simulink model "test_td"  (R2022b)
settings: Solver=VariableStepAuto  StartTime=0.0  StopTime=10  RelTol=1e-3
undefined symbols (not defined in the file or in its folder): den, num
libraries: simulink x2, slpidlib x1, dspsrcs4 x1
settings Model: Creator=张倬境  LastModifiedBy=张倬境

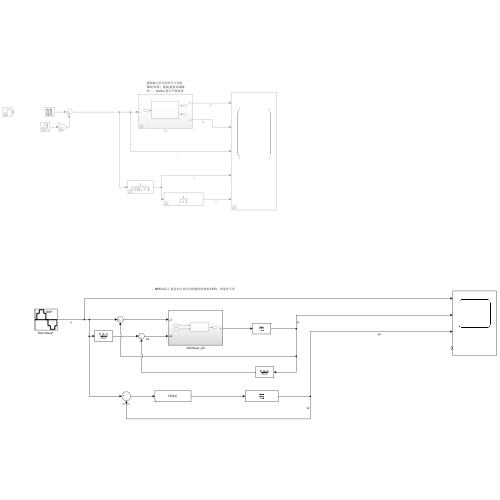
[thumbnail: Simulink's stored preview of the top-level diagram]
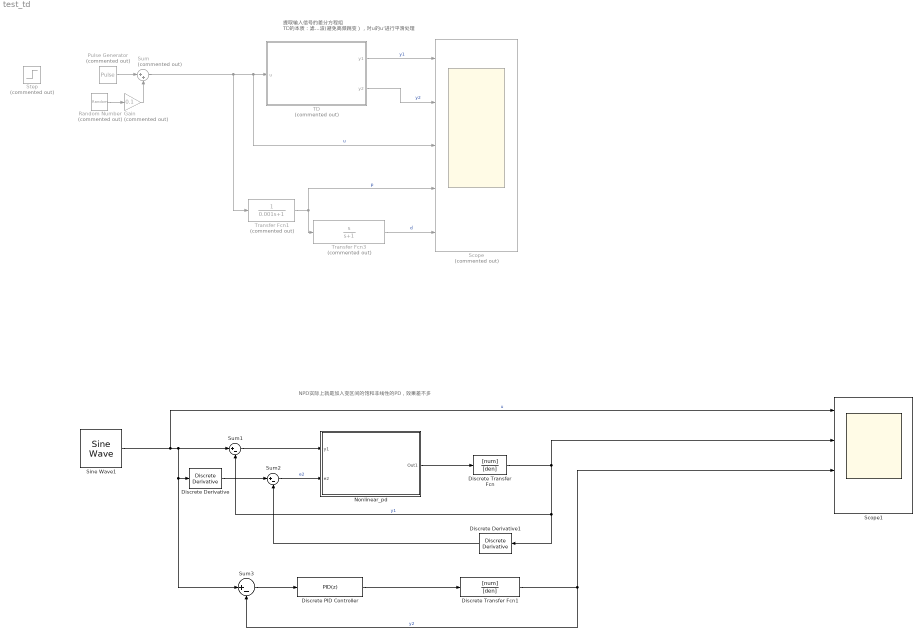
== system test_td ==
  note: NPD实际上就是加入变区间的饱和非线性的PD，效果差不多
  note: 提取输入信号的差分方程组
      | TD的本质：滤波(避免高频跳变），对u的u‘进行平滑处理
  Discrete Transfer Fcn : DiscreteTransferFcn  Numerator=[num]  Denominator=[den]
  Discrete Transfer Fcn1 : DiscreteTransferFcn  Numerator=[num]  Denominator=[den]
  Discrete Derivative : simulink/Discrete/Discrete Derivative  gainval=1.0  ICPrevScaledInput=0.0  OutMin=[]  OutMax=[]  OutDataType=fixdt(1, 16)  OutScaling=2^-10  DoSatur=off
  Discrete Derivative1 : simulink/Discrete/Discrete Derivative  gainval=1.0  ICPrevScaledInput=0.0  OutMin=[]  OutMax=[]  OutDataType=fixdt(1, 16)  OutScaling=2^-10  DoSatur=off
  Discrete PID Controller : slpidlib/PID Controller  Controller=PID  Form=Parallel  TimeDomain=Discrete-time  UseExternalTs=off  SampleTime=-1  IntegratorMethod=Forward Euler  FilterMethod=Forward Euler  ControllerParametersSource=internal  P=100  I=0  UseKiTs=off  D=0  N=10  UseFilter=off  TunerSelectOption=Frequency Response Based  InitialConditionSource=internal  InitialConditionForIntegrator=0  InitialConditionForFilter=0  DifferentiatorICPrevScaledInput=0  ExternalReset=none  TrackingMode=off  Kt=1  LimitOutput=off  SatLimitsSource=internal  UpperSaturationLimit=inf  LowerSaturationLimit=-inf  LinearizeAsGain=off  AntiWindupMode=none  Kb=1  LimitIntegrator=off  UpperIntegratorSaturationLimit=inf  LowerIntegratorSaturationLimit=-inf  POutMin=[]  POutMax=[]  IOutMin=[]  IOutMax=[]  DOutMin=[]  DOutMax=[]  NOutMin=[]  NOutMax=[]  SumOutMin=[]  SumOutMax=[]  SaturationOutMin=[]  SaturationOutMax=[]  PParamMin=[]  PParamMax=[]  IParamMin=[]  IParamMax=[]  DParamMin=[]  DParamMax=[]  NParamMin=[]  NParamMax=[]  KbParamMin=[]  KbParamMax=[]  KtParamMin=[]  KtParamMax=[]  KbOutMin=[]  KbOutMax=[]  KtOutMin=[]  KtOutMax=[]  IntegratorOutMin=[]  IntegratorOutMax=[]  FilterOutMin=[]  FilterOutMax=[]  SumI1OutMin=[]  SumI1OutMax=[]  SumI2OutMin=[]  SumI2OutMax=[]  SumI3OutMin=[]  SumI3OutMax=[]  SumI4OutMin=[]  SumI4OutMax=[]  SumDOutMin=[]  SumDOutMax=[]  DifferentiatorOutMin=[]  DifferentiatorOutMax=[]  FilterDiffOutCoefMin=[]  FilterDiffOutCoefMax=[]  ReciprocalOutMin=[]  ReciprocalOutMax=[]  SumDenOutMin=[]  SumDenOutMax=[]  SumNumOutMin=[]  SumNumOutMax=[]  DivideOutMin=[]  DivideOutMax=[]  UdiffTsProdOutMin=[]  UdiffTsProdOutMax=[]  NTsProdOutMin=[]  NTsProdOutMax=[]  UintegralTsProdOutMin=[]  UintegralTsProdOutMax=[]  UngainTsProdOutMin=[]  UngainTsProdOutMax=[]  ClampingZeroOutDataTypeStr=Inherit: Inherit via back propagation  ClampingZeroOutMin=[]  ClampingZeroOutMax=[]  FilterDenConstantOutDataTypeStr=Inherit: Inherit via back propagation  FilterDenConstantOutMin=[]  FilterDenConstantOutMax=[]  PCopyOutDataTypeStr=Inherit: Inherit via back propagation  PCopyOutMin=[]  PCopyOutMax=[]  NCopyOutDataTypeStr=Inherit: Inherit via back propagation  NCopyOutMin=[]  NCopyOutMax=[]  IntegratorContinuousStateAttributes=''  IntegratorStateMustResolveToSignalObject=off  IntegratorRTWStateStorageClass=Auto  FilterContinuousStateAttributes=''  FilterStateMustResolveToSignalObject=off  FilterRTWStateStorageClass=Auto  ParallelPVariant=InternalParameters  IdealPVariant=Disabled  IVariant=InternalParameters  DVariant=InternalParameters  IntegratorVariant=Discrete  SatVariant=Disabled  AWVariant=Passthrough  PCopyVariant=Disabled  TRVariant=Disabled  FdbkBlocksVariant=Forward  IdealPFdbkVariant=Disabled  SatFdbkVariant=Disabled  DerivativeFilterVariant=Differentiator  NVariant=Passthrough  NCopyVariant=Disabled_SignalSpec  FilterICVariant=InternalICsDifferentiator  IntegratorICVariant=InternalICs  ExternalResetVariant=Disabled  TRSumVariant=Passthrough  SumFdbkVariant=Disabled  SumVariant=Sum_PID  TsampFilterVariant=InternalTs  TsampNgainVariant=Passthrough  TsampIntegralVariant=Passthrough  ExternalSaturationOutDataTypeStr=Inherit: Same as second input
      settings: LibrarySourceBlock=simulink/Discrete/Discrete PID Controller
  Gain : Gain  Commented=on  Gain=0.1
  Nonlinear_pd : Subsystem
  Pulse Generator : DiscretePulseGenerator  Commented=on  PulseType=Time based  Period=4  PulseWidth=50
  Random Number : RandomNumber  Commented=on  Variance=0.01  SampleTime=0.1
  Scope : Scope  Commented=on  NumInputPorts=5
  Scope1 : Scope  NumInputPorts=4
  Sine Wave1 : dspsrcs4/Sine Wave  Amplitude=1  Frequency=1/4  Phase=0  SampleMode=Discrete  OutComplex=Real  CompMethod=Trigonometric fcn  TableSize=Speed  SampleTime=1/100  SamplesPerFrame=1  ResetState=Restart at time zero  OutputFrames=off  dataType=double  wordLen=16  udDataType=sfix(16)  fracBitsMode=Best precision  numFracBits=15  OutDataTypeStr=double  LastOutDataTypeStr=double
  Step : Step  Commented=on  SampleTime=0
  Sum : Sum  Commented=on  Inputs=|++
  Sum1 : Sum  Inputs=|+-
  Sum2 : Sum  Inputs=|+-
  Sum3 : Sum  Inputs=|+-
  TD : Subsystem  Commented=on
  Transfer Fcn1 : TransferFcn  Commented=on  Denominator=[0.001 1]
  Transfer Fcn3 : TransferFcn  Commented=on  Numerator=[1 0]  Denominator=[1 1]
  wires:
  Sum/1 -> Transfer Fcn1/1, Scope/3, TD/1(u)  "u"
  Random Number/1 -> Gain/1
  Gain/1 -> Sum/2
  TD/1(y1) -> Scope/1  "y1"
  Transfer Fcn1/1 -> Scope/4, Transfer Fcn3/1  "p"
  TD/2(y2) -> Scope/2  "y2"
  Transfer Fcn3/1 -> Scope/5  "d"
  Pulse Generator/1 -> Sum/1
  Sum1/1 -> Nonlinear_pd/1(y1)
  Sum2/1 -> Nonlinear_pd/2(e2)  "e2"
  Sine Wave1/1 -> Scope1/1, Sum3/1, Discrete Derivative/1, Sum1/1  "u"
  Nonlinear_pd/1(Out1) -> Discrete Transfer Fcn/1
  Discrete Transfer Fcn/1 -> Discrete Derivative1/1, Sum1/2, Scope1/2  "y1"
  Discrete Derivative1/1 -> Sum2/2
  Discrete Derivative/1 -> Sum2/1
  Sum3/1 -> Discrete PID Controller/1
  Discrete PID Controller/1 -> Discrete Transfer Fcn1/1
  Discrete Transfer Fcn1/1 -> Sum3/2, Scope1/3  "y2"

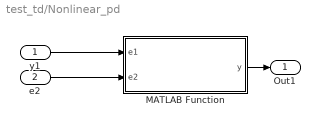
== system test_td/Nonlinear_pd ==
  y1 : Inport
  e2 : Inport  Port=2
  MATLAB Function : MATLAB Function  TreatAsAtomicUnit=on
  Out1 : Outport
  wires:
  y1/1 -> MATLAB Function/1(e1)
  MATLAB Function/1(y) -> Out1/1
  e2/1 -> MATLAB Function/2(e2)

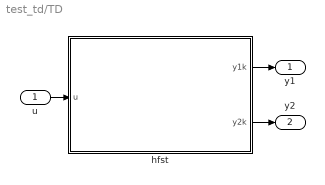
== system test_td/TD ==
  u : Inport
  hfst : MATLAB Function  TreatAsAtomicUnit=on  SystemSampleTime=0.01
  y1 : Outport
  y2 : Outport  Port=2
  wires:
  u/1 -> hfst/1(u)
  hfst/1(y1k) -> y1/1
  hfst/2(y2k) -> y2/1

== matlab function test_td/TD/hfst ==
  data: u input; y1k output; y2k output
function [y1k,y2k] = fcn(u)
persistent y1k_1 y2k_1
h=0.01;
delta=10;
if isempty(y1k_1)
    y1k_1=0;
end


if isempty(y2k_1)
    y2k_1=0;
end


y1k=y1k_1+h*y2k_1;


% hfst计算内容
d=delta*h;
d0=h*d;
y=y1k_1-u+h*y2k_1;
a0=sqrt(d*d+8*delta*abs(y));
a=0;
out1=0;
if abs(y)>d0
    a=y2k_1+(a0-d)/2*sign(y);
end


if abs(y)<=d0
    a=y2k_1+y/h;
end


if abs(a)>d
    out1=-delta*sign(a);
end


if abs(a)<=d
    out1=-delta*a/d;
end
out=out1;
% 更新变量
y2k=y2k_1+h*out;


y1k_1=y1k;
y2k_1=y2k;


end

== matlab function test_td/Nonlinear_pd/MATLAB Function ==
  data: e1 input; y output; e2 input
function y =nonlinear_pd(e1,e2)
alfa1=0.75;
alfa2=1.5;
delta=0.5;
beta1=100;
beta2=1;
fal1=1;
fal2=1;


if abs(e1)<=delta
    fal1=e1/(delta^(1-alfa1));
end


if abs(e1)>delta
    fal1=(abs(e1))^(alfa1)*sign(e1);
end


if abs(e2)<=delta
    fal2=e2/(delta^(1-alfa2));
end


if abs(e2)>delta
    fal2=(abs(e2))^(alfa2)*sign(e2);
end


y=beta1*fal1+beta2*fal2;
end
